simulink subsystem "VCU"  (R2023b)
settings: Solver=VariableStepAuto  StartTime=0.0  StopTime=10.0  RelTol=1e-3
values from neighbouring files (symbols this model uses):
  UC_State = <binary blob, 1881 chars, not shown>    [rev3_data.sldd]
settings Model: Creator=mjmag  LastModifiedBy=mjmag

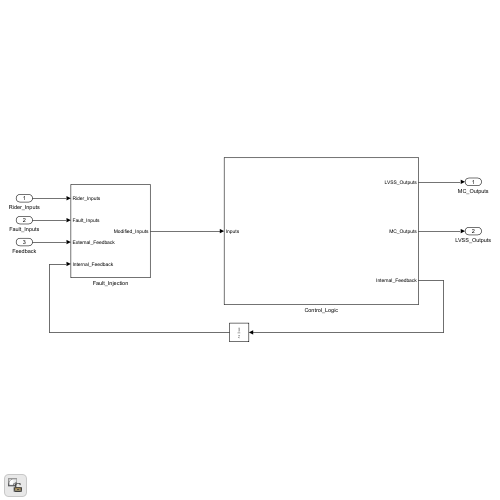
[thumbnail: Simulink's stored preview of the top-level diagram]
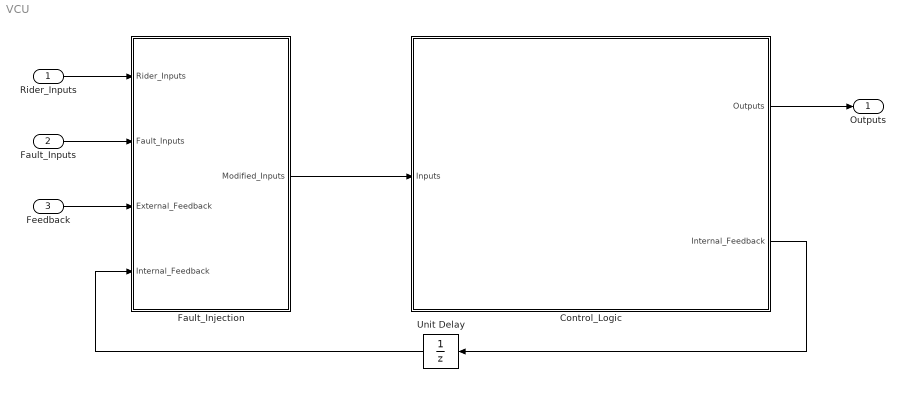
== system VCU ==
  Rider_Inputs : Inport
  Fault_Inputs : Inport  Port=2
  Feedback : Inport  Port=3
  Control_Logic : Subsystem
  Fault_Injection : Subsystem
  Unit Delay : UnitDelay  SampleTime=-1  HasFrameUpgradeWarning=on
  Outputs : Outport
  wires:
  Fault_Injection/1(Modified_Inputs) -> Control_Logic/1(Inputs)
  Fault_Inputs/1 -> Fault_Injection/2(Fault_Inputs)
  Control_Logic/2(Internal_Feedback) -> Unit Delay/1
  Rider_Inputs/1 -> Fault_Injection/1(Rider_Inputs)
  Feedback/1 -> Fault_Injection/3(External_Feedback)
  Unit Delay/1 -> Fault_Injection/4(Internal_Feedback)
  Control_Logic/1(Outputs) -> Outputs/1

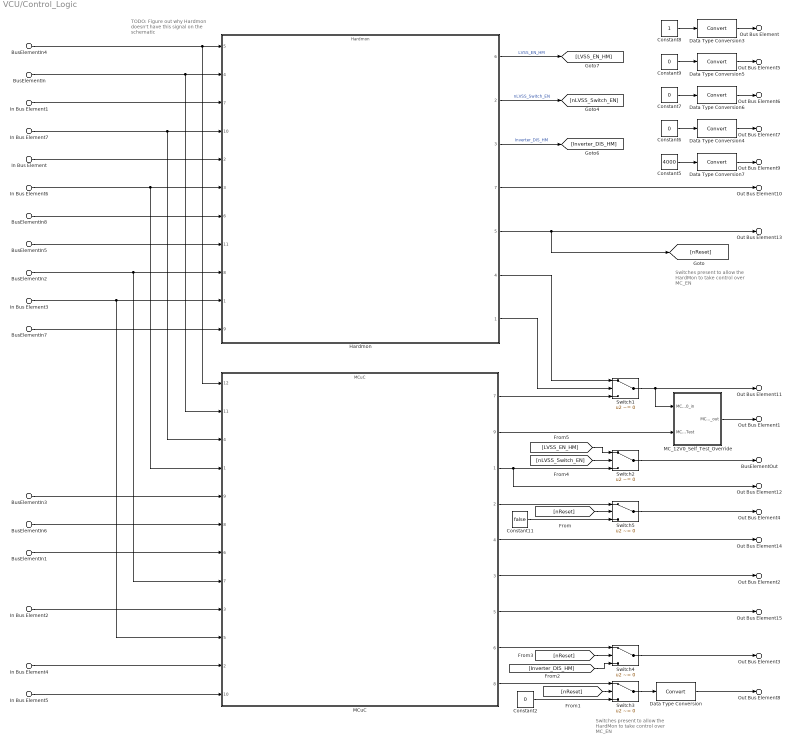
== system VCU/Control_Logic ==
  note: Switches present to allow the HardMon to take control over MC_EN
  note: Switches present to allow the HardMon to take control over MC_EN
  note: TODO: Figure out why Hardmon doesn't have this signal on the schematic
  In Bus Element : Inport  PortName=Inputs  Element=Rider_Inputs.Key_In.LS_B
  In Bus Element6 : Inport  PortName=Inputs  Element=Rider_Inputs.Key_In.LS_A
  In Bus Element1 : Inport  PortName=Inputs  Element=Rider_Inputs.Estop_In.LS_B
  In Bus Element7 : Inport  PortName=Inputs  Element=Rider_Inputs.Estop_In.LS_A
  In Bus Element2 : Inport  PortName=Inputs  Element=Rider_Inputs.Brake
  In Bus Element3 : Inport  PortName=Inputs  Element=Rider_Inputs.Forward_EN
  In Bus Element4 : Inport  PortName=Inputs  Element=Rider_Inputs.Start
  In Bus Element5 : Inport  PortName=Inputs  Element=Rider_Inputs.Throttle
  BusElementIn : Inport  PortName=Inputs  Element=Feedback.LVSS_Feedback.LVSS_ON
  BusElementIn1 : Inport  PortName=Inputs  Element=Feedback.MC_Feedback.D1_VSM_State
  BusElementIn2 : Inport  PortName=Inputs  Element=Feedback.MC_Feedback.D4_Inverter_Discharge_State
  BusElementIn3 : Inport  PortName=Inputs  Element=Feedback.Internal_Feedback.HM_Fault
  BusElementIn4 : Inport  PortName=Inputs  Element=Feedback.Internal_Feedback.MC_12V0
  BusElementIn5 : Inport  PortName=Inputs  Element=Feedback.Internal_Feedback.LVSS_EN_uC
  BusElementIn6 : Inport  PortName=Inputs  Element=Feedback.Internal_Feedback.nReset
  BusElementIn7 : Inport  PortName=Inputs  Element=Feedback.Internal_Feedback.Watchdog
  BusElementIn8 : Inport  PortName=Inputs  Element=Feedback.Internal_Feedback.uC_State
  Constant11 : Constant  Value=false
  Constant{2,6..7,9} (4 alike) : Constant  Value=0
  Constant5 : Constant  Value=4000
  Constant8 : Constant
  Data Type Conversion : DataTypeConversion  OutMin=[-32768]  OutMax=[32767]  SaturateOnIntegerOverflow=off  RndMeth=Floor
  Data Type Conversion{3..7} (5 alike) : DataTypeConversion  SaturateOnIntegerOverflow=off  RndMeth=Floor
  Hardmon : ModelReference  ModelNameDialog=Hardmon  SimulationMode=Normal  ModelReferenceVersion=1.66
      settings: PortSchema="{\"entries\":[{\"content\":{\"sides\":[{\"content\":{\"connectorIds\":[\"In5\",\"In4\",\"In7\",\"In10\",\"In2\",\"In3\",\"In6\",\"In11\",\"In8\",\"In1\",\"In9\"]},\"type\":\"ConnectorPlacement.EquallySpacedRectSide\",\"uuid\":\"ce77178b-c7f8-493e-81d6-6e6e47cbf042\"},{\"content\":{\"connectorIds\":[\"Out6\",\"Out2\",\"Out3\",\"Out7\",\"Out5\",\"Out4\",\"Out1\"],\"side\":\"RIGHT\"},\"type\":\"ConnectorPlacement.EquallySpacedRectSide\",\"uuid\":\"9ebffa51-7eff-4dd8-ac2f-4fbc962f2290\"},{\"content\":{\"side\":\"TOP\"},\"type\":\"ConnectorPlacement.EquallySpacedRectSide\",\"uuid\":\"a2dadd06-97c4-4e35-990a-e30edfa10790\"},{\"content\":{\"side\":\"BOTTOM\"},\"type\":\"ConnectorPlacement.EquallySpacedRectSide\",\"uuid\":\"517832bd-7eeb-47f8-b142-e0ae288b30eb\"}]},\"type\":\"ConnectorPlacement.EquallySpacedConnector\",\"uuid\":\"ad9c7ae8-ba7b-4478-b44d-db7efe0b7c30\"}],\"packageUris\":[\"http://schema.mathworks.com/mf0/Connector/R2020b\"],\"version\":\"1.0\"}"
  MC_12V0_Self_Test_Override : Subsystem
  MCuC : ModelReference  ModelNameDialog=MCuC.slx  SimulationMode=Normal  ModelReferenceVersion=1.17
      settings: PortSchema="{\"entries\":[{\"content\":{\"sides\":[{\"content\":{\"connectorIds\":[\"In12\",\"In11\",\"In4\",\"In1\",\"In9\",\"In8\",\"In6\",\"In7\",\"In3\",\"In5\",\"In2\",\"In10\"]},\"type\":\"ConnectorPlacement.EquallySpacedRectSide\",\"uuid\":\"29930030-cffb-426b-9232-13bdddb5f01a\"},{\"content\":{\"connectorIds\":[\"Out7\",\"Out9\",\"Out1\",\"Out2\",\"Out4\",\"Out3\",\"Out5\",\"Out6\",\"Out8\"],\"side\":\"RIGHT\"},\"type\":\"ConnectorPlacement.EquallySpacedRectSide\",\"uuid\":\"e039672f-acfd-4e0d-841a-f9c7cf53404a\"},{\"content\":{\"side\":\"TOP\"},\"type\":\"ConnectorPlacement.EquallySpacedRectSide\",\"uuid\":\"ed3172ff-ca70-451f-85df-845f56faf5b0\"}]},\"type\":\"ConnectorPlacement.EquallySpacedConnector\",\"uuid\":\"b36a8819-9044-4231-aae1-023be34ba1c8\"}],\"packageUris\":[\"http://schema.mathworks.com/mf0/Connector/R2020b\"],\"version\":\"1.0\"}"
  Switch{1..5} (5 alike) : Switch  Criteria=u2 ~= 0  SaturateOnIntegerOverflow=off  InputSameDT=off
  Out Bus Element : Outport  PortName=Outputs  Element=MC_Outputs.MC_Command.Direction_Command
  Out Bus Element5 : Outport  PortName=Outputs  Element=MC_Outputs.MC_Command.Rolling_Counter
  Out Bus Element6 : Outport  PortName=Outputs  Element=MC_Outputs.MC_Command.Speed_Command
  Out Bus Element7 : Outport  PortName=Outputs  Element=MC_Outputs.MC_Command.Speed_Mode_Enable
  Out Bus Element9 : Outport  PortName=Outputs  Element=MC_Outputs.MC_Command.Torque_Limit_Command
  Out Bus Element4 : Outport  PortName=Outputs  Element=MC_Outputs.MC_Command.Inverter_Enable
  Out Bus Element3 : Outport  PortName=Outputs  Element=MC_Outputs.MC_Command.Inverter_Discharge
  Out Bus Element8 : Outport  PortName=Outputs  Element=MC_Outputs.MC_Command.Torque_Command
  Out Bus Element1 : Outport  PortName=Outputs  Element=MC_Outputs.MC_12V0
  Out Bus Element2 : Outport  PortName=Outputs  Element=MC_Outputs.Fault_To_MC
  BusElementOut : Outport  PortName=Outputs  Element=LVSS_Outputs.LVSS_EN
  Out Bus Element10 : Outport  Port=2  PortName=Internal_Feedback  Element=HM_Fault
  Out Bus Element11 : Outport  Port=2  PortName=Internal_Feedback  Element=MC_12V0
  Out Bus Element12 : Outport  Port=2  PortName=Internal_Feedback  Element=LVSS_EN_uC
  Out Bus Element13 : Outport  Port=2  PortName=Internal_Feedback  Element=nReset
  Out Bus Element14 : Outport  Port=2  PortName=Internal_Feedback  Element=Watchdog
  Out Bus Element15 : Outport  Port=2  PortName=Internal_Feedback  Element=uC_State
  wires:
  Data Type Conversion7/1 -> Out Bus Element9/1
  Data Type Conversion6/1 -> Out Bus Element6/1
  Data Type Conversion5/1 -> Out Bus Element5/1
  Data Type Conversion4/1 -> Out Bus Element7/1
  Data Type Conversion3/1 -> Out Bus Element/1
  BusElementIn2/1 -> MCuC/7, Hardmon/8
  BusElementIn1/1 -> MCuC/6
  Switch2/1 -> BusElementOut/1
  MCuC/5 -> Out Bus Element15/1
  Switch1/1 -> Out Bus Element11/1, MC_12V0_Self_Test_Override/1(MC_12V0_in)
  Constant5/1 -> Data Type Conversion7/1
  Constant8/1 -> Data Type Conversion3/1
  In Bus Element3/1 -> MCuC/5, Hardmon/1
  In Bus Element6/1 -> MCuC/1, Hardmon/3
  In Bus Element7/1 -> MCuC/4, Hardmon/10
  Hardmon/6 -> [LVSS_EN_HM]  "LVSS_EN_HM"
  [Inverter_DIS_HM] -> Switch4/3
  MCuC/3 -> Out Bus Element2/1
  Hardmon/2 -> [nLVSS_Switch_EN]  "nLVSS_Switch_EN"
  Data Type Conversion/1 -> Out Bus Element8/1
  In Bus Element4/1 -> MCuC/2
  Constant7/1 -> Data Type Conversion6/1
  Constant11/1 -> Switch5/3
  Hardmon/1 -> Switch1/2
  [nReset] -> Switch5/2
  BusElementIn4/1 -> MCuC/12, Hardmon/5
  BusElementIn5/1 -> Hardmon/11
  Constant9/1 -> Data Type Conversion5/1
  BusElementIn7/1 -> Hardmon/9
  MCuC/9 -> MC_12V0_Self_Test_Override/2(MC_Self_Test)
  In Bus Element2/1 -> MCuC/3
  BusElementIn8/1 -> Hardmon/6
  Switch5/1 -> Out Bus Element4/1
  Hardmon/3 -> [Inverter_DIS_HM]  "Inverter_DIS_HM"
  Constant2/1 -> Switch3/3
  BusElementIn/1 -> MCuC/11, Hardmon/4
  MCuC/1 -> Switch2/3, Out Bus Element12/1
  In Bus Element/1 -> Hardmon/2
  MCuC/2 -> Switch5/1
  BusElementIn3/1 -> MCuC/9
  MCuC/4 -> Out Bus Element14/1
  MCuC/7 -> Switch1/3
  In Bus Element1/1 -> Hardmon/7
  Switch3/1 -> Data Type Conversion/1
  BusElementIn6/1 -> MCuC/8
  [nLVSS_Switch_EN] -> Switch2/2
  MCuC/8 -> Switch3/1
  Hardmon/5 -> Out Bus Element13/1, [nReset]
  [LVSS_EN_HM] -> Switch2/1
  Constant6/1 -> Data Type Conversion4/1
  Switch4/1 -> Out Bus Element3/1
  In Bus Element5/1 -> MCuC/10
  [nReset] -> Switch3/2
  Hardmon/7 -> Out Bus Element10/1
  [nReset] -> Switch4/2
  MCuC/6 -> Switch4/1
  MC_12V0_Self_Test_Override/1(MC_12V0_out) -> Out Bus Element1/1
  Hardmon/4 -> Switch1/1

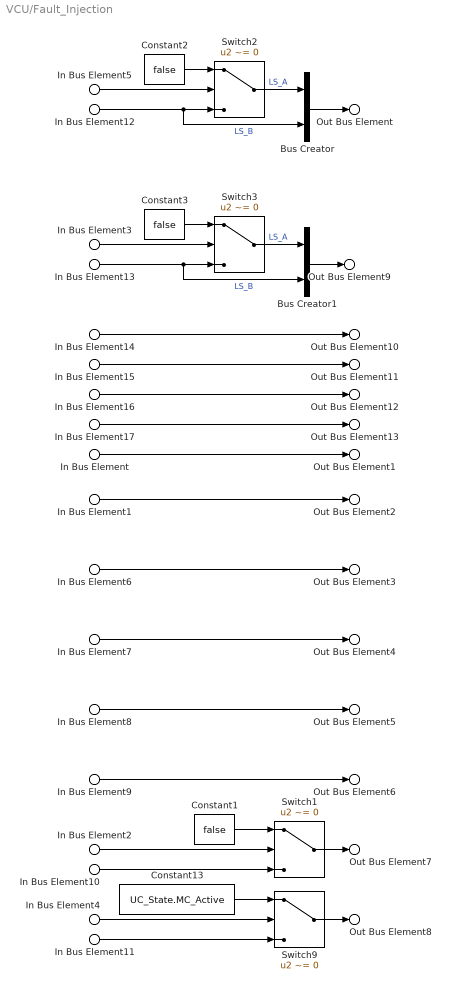
== system VCU/Fault_Injection ==
  In Bus Element12 : Inport  PortName=Rider_Inputs  Element=Key_In
  In Bus Element13 : Inport  PortName=Rider_Inputs  Element=Estop_In
  In Bus Element14 : Inport  PortName=Rider_Inputs  Element=Brake
  In Bus Element15 : Inport  PortName=Rider_Inputs  Element=Forward_EN
  In Bus Element16 : Inport  PortName=Rider_Inputs  Element=Start
  In Bus Element17 : Inport  PortName=Rider_Inputs  Element=Throttle
  In Bus Element2 : Inport  Port=2  PortName=Fault_Inputs  Element=Force_WD_Low
  In Bus Element3 : Inport  Port=2  PortName=Fault_Inputs  Element=Force_Estop_Low
  In Bus Element4 : Inport  Port=2  PortName=Fault_Inputs  Element=Force_UC_State_3
  In Bus Element5 : Inport  Port=2  PortName=Fault_Inputs  Element=Force_Ignition_High
  In Bus Element : Inport  Port=3  PortName=External_Feedback  Element=MC_Feedback
  In Bus Element1 : Inport  Port=3  PortName=External_Feedback  Element=LVSS_Feedback
  In Bus Element6 : Inport  Port=4  PortName=Internal_Feedback  Element=HM_Fault
  In Bus Element7 : Inport  Port=4  PortName=Internal_Feedback  Element=MC_12V0
  In Bus Element8 : Inport  Port=4  PortName=Internal_Feedback  Element=LVSS_EN_uC
  In Bus Element9 : Inport  Port=4  PortName=Internal_Feedback  Element=nReset
  In Bus Element10 : Inport  Port=4  PortName=Internal_Feedback  Element=Watchdog
  In Bus Element11 : Inport  Port=4  PortName=Internal_Feedback  Element=uC_State
  Bus Creator : BusCreator  Inputs=2
  Bus Creator1 : BusCreator  Inputs=2
  Constant1 : Constant  Value=false  OutDataTypeStr=Inherit: Inherit via back propagation
  Constant13 : Constant  Value=UC_State.MC_Active  OutDataTypeStr=Inherit: Inherit via back propagation
  Constant2 : Constant  Value=false  OutDataTypeStr=Inherit: Inherit via back propagation
  Constant3 : Constant  Value=false  OutDataTypeStr=Inherit: Inherit via back propagation
  Switch{1..3,9} (4 alike) : Switch  Criteria=u2 ~= 0  OutDataTypeStr=Inherit: Inherit via back propagation  SaturateOnIntegerOverflow=off  InputSameDT=off
  Out Bus Element : Outport  PortName=Modified_Inputs  Element=Rider_Inputs.Key_In
  Out Bus Element9 : Outport  PortName=Modified_Inputs  Element=Rider_Inputs.Estop_In
  Out Bus Element10 : Outport  PortName=Modified_Inputs  Element=Rider_Inputs.Brake
  Out Bus Element11 : Outport  PortName=Modified_Inputs  Element=Rider_Inputs.Forward_EN
  Out Bus Element12 : Outport  PortName=Modified_Inputs  Element=Rider_Inputs.Start
  Out Bus Element13 : Outport  PortName=Modified_Inputs  Element=Rider_Inputs.Throttle
  Out Bus Element1 : Outport  PortName=Modified_Inputs  Element=Feedback.MC_Feedback
  Out Bus Element2 : Outport  PortName=Modified_Inputs  Element=Feedback.LVSS_Feedback
  Out Bus Element3 : Outport  PortName=Modified_Inputs  Element=Feedback.Internal_Feedback.HM_Fault
  Out Bus Element4 : Outport  PortName=Modified_Inputs  Element=Feedback.Internal_Feedback.MC_12V0
  Out Bus Element5 : Outport  PortName=Modified_Inputs  Element=Feedback.Internal_Feedback.LVSS_EN_uC
  Out Bus Element6 : Outport  PortName=Modified_Inputs  Element=Feedback.Internal_Feedback.nReset
  Out Bus Element7 : Outport  PortName=Modified_Inputs  Element=Feedback.Internal_Feedback.Watchdog
  Out Bus Element8 : Outport  PortName=Modified_Inputs  Element=Feedback.Internal_Feedback.uC_State
  wires:
  In Bus Element13/1 -> Switch3/3, Bus Creator1/2  "LS_B"
  Bus Creator1/1 -> Out Bus Element9/1
  Constant3/1 -> Switch3/1
  Switch3/1 -> Bus Creator1/1  "LS_A"
  In Bus Element3/1 -> Switch3/2
  In Bus Element5/1 -> Switch2/2
  Switch2/1 -> Bus Creator/1  "LS_A"
  Constant2/1 -> Switch2/1
  Bus Creator/1 -> Out Bus Element/1
  In Bus Element17/1 -> Out Bus Element13/1
  In Bus Element16/1 -> Out Bus Element12/1
  In Bus Element15/1 -> Out Bus Element11/1
  In Bus Element14/1 -> Out Bus Element10/1
  In Bus Element12/1 -> Switch2/3, Bus Creator/2  "LS_B"
  In Bus Element2/1 -> Switch1/2
  Switch1/1 -> Out Bus Element7/1
  Constant1/1 -> Switch1/1
  Switch9/1 -> Out Bus Element8/1
  Constant13/1 -> Switch9/1
  In Bus Element4/1 -> Switch9/2
  In Bus Element11/1 -> Switch9/3
  In Bus Element10/1 -> Switch1/3
  In Bus Element9/1 -> Out Bus Element6/1
  In Bus Element8/1 -> Out Bus Element5/1
  In Bus Element7/1 -> Out Bus Element4/1
  In Bus Element6/1 -> Out Bus Element3/1
  In Bus Element1/1 -> Out Bus Element2/1
  In Bus Element/1 -> Out Bus Element1/1

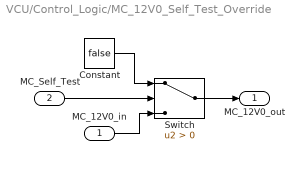
== system VCU/Control_Logic/MC_12V0_Self_Test_Override ==
  MC_12V0_in : Inport
  MC_Self_Test : Inport  Port=2
  Constant : Constant  Value=false
  Switch : Switch  Criteria=u2 > Threshold  SaturateOnIntegerOverflow=off  InputSameDT=off
  MC_12V0_out : Outport
  wires:
  MC_12V0_in/1 -> Switch/3
  Constant/1 -> Switch/1
  Switch/1 -> MC_12V0_out/1
  MC_Self_Test/1 -> Switch/2
